simulink model "Exercise_6_1"  (R2024b)
settings: Solver=VariableStepAuto  StartTime=0.0  StopTime=10000  RelTol=1e-3
undefined symbols (not defined in the file): alpha, eta, I_tot, k_q, N
settings Model: Creator=lukas  LastModifiedBy=lukas

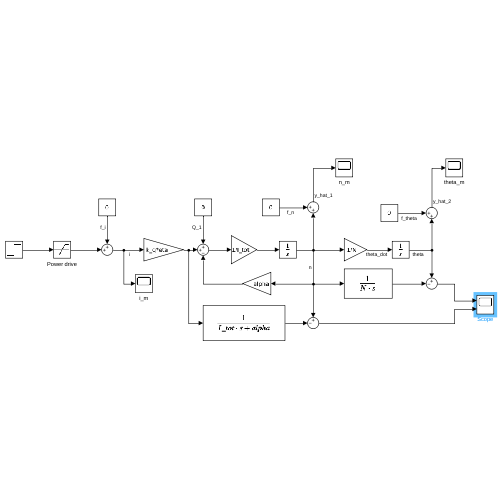
[thumbnail: Simulink's stored preview of the top-level diagram]
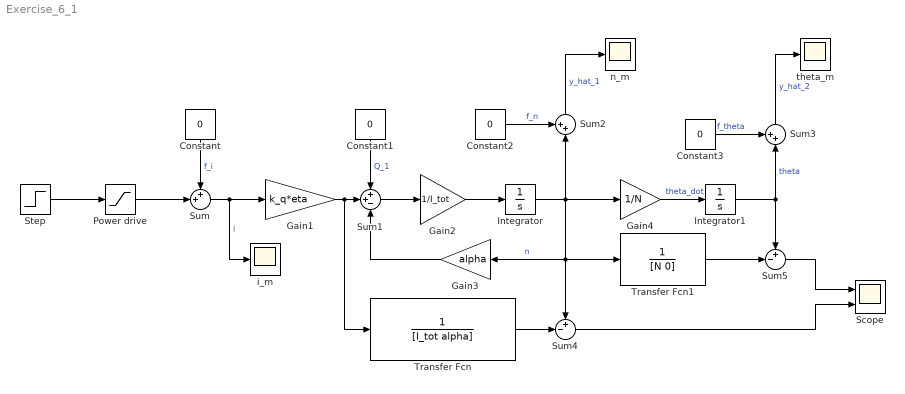
== system Exercise_6_1 ==
  Constant{,1..3} (4 alike) : Constant  Value=0
  Gain1 : Gain  Gain=k_q*eta
  Gain2 : Gain  Gain=1/I_tot
  Gain3 : Gain  Gain=alpha
  Gain4 : Gain  Gain=1/N
  Integrator : Integrator
  Integrator1 : Integrator
  Power drive : Saturate
  Scope : Scope  NumInputPorts=2
  Step : Step  SampleTime=0
  Sum : Sum  Inputs=++|
  Sum1 : Sum  Inputs=++-
  Sum2 : Sum  Inputs=++|
  Sum3 : Sum  Inputs=++|
  Sum4 : Sum  Inputs=+-|
  Sum5 : Sum  Inputs=+-|
  Transfer Fcn : TransferFcn  Denominator=[I_tot alpha]
  Transfer Fcn1 : TransferFcn  Denominator=[N 0]
  i_m : Scope
  n_m : Scope
  theta_m : Scope
  wires:
  Power drive/1 -> Sum/2
  Sum/1 -> i_m/1, Gain1/1  "i"
  Gain1/1 -> Transfer Fcn/1, Sum1/2
  Sum1/1 -> Gain2/1
  Gain2/1 -> Integrator/1
  Gain3/1 -> Sum1/3
  Integrator/1 -> Gain4/1, Sum4/1, Transfer Fcn1/1, Gain3/1, Sum2/2  "n"
  Gain4/1 -> Integrator1/1  "theta_dot"
  Constant1/1 -> Sum1/1  "Q_1"
  Step/1 -> Power drive/1
  Constant/1 -> Sum/1  "f_i"
  Constant2/1 -> Sum2/1  "f_n"
  Sum2/1 -> n_m/1  "y_hat_1"
  Integrator1/1 -> Sum5/1, Sum3/2  "theta"
  Sum3/1 -> theta_m/1  "y_hat_2"
  Constant3/1 -> Sum3/1  "f_theta"
  Transfer Fcn/1 -> Sum4/2
  Sum4/1 -> Scope/2
  Transfer Fcn1/1 -> Sum5/2
  Sum5/1 -> Scope/1
